simulink model "joystick_ctrl"  (Simulink 6.4)
settings: Solver=FixedStepDiscrete  SolverMode=SingleTasking  StartTime=0  StopTime=inf  FixedStep=0.001  RelTol=1e-3
PreLoadFcn:
  | load_logdata;
  | SoundList;
libraries: ecrobot_nxt_lib x10, simulink x4
CloseFcn:
  | rtwprivate ssgencode ModelCloseRequest TestBluetooth
settings Model: Creator=banno  LastModifiedBy=tchikama  CovPath=/Joystick_app  CovMetricSettings=dcmtrw  ProdHWDeviceType=ARM7
settings DataIOCC: SaveOutput=off  SignalLogging=off  SaveTime=off
settings OptimizationCC: InlineParams=on  InlineInvariantSignals=on  RollThreshold=2  StateBitsets=on  DataBitsets=on  UseTempVars=on  InitFltsAndDblsToZero=off  NoFixptDivByZeroProtection=on  EfficientFloat2IntCast=on  OptimizeModelRefInitCode=on  LifeSpan=1
settings DebuggingCC: ConsistencyChecking=warning  SignalInfNanChecking=warning  ReadBeforeWriteMsg=DisableAll  WriteAfterWriteMsg=DisableAll  WriteAfterReadMsg=DisableAll  AlgebraicLoopMsg=error  CheckExecutionContextPreStartOutputMsg=on  CheckExecutionContextRuntimeOutputMsg=on  SolverPrmCheckMsg=none  SingleTaskRateTransMsg=warning  TasksWithSamePriorityMsg=none  IntegerOverflowMsg=error  ParameterPrecisionLossMsg=none  UnconnectedInputMsg=error  UnconnectedOutputMsg=error  UnconnectedLineMsg=error  UniqueDataStoreMsg=error  BusObjectLabelMismatch=error  RootOutportRequireBusObject=error  ModelReferenceIOMsg=warning  ModelReferenceVersionMismatchMessage=warning  ModelReferenceIOMismatchMessage=warning
settings HardwareCC: ProdIntDivRoundTo=Zero  ProdEndianess=LittleEndian  ProdHWDeviceType=ARM7  TargetHWDeviceType=32-bit Generic
settings ModelReferenceCC: ModelReferenceNumInstancesAllowed=Single
settings RTWCC: SystemTargetFile=ert.tlc  GenCodeOnly=on  GenerateMakefile=off  TemplateMakefile=ert_default_tmf  Description=Real-Time Workshop Embedded Coder (no auto configuration)  GenerateReport=on  RTWVerbose=off  ProcessScript=ert_make_rtw_hook  IncludeHyperlinkInReport=on  LaunchReport=on
settings CodeAppCC: ForceParamTrailComments=on  IgnoreCustomStorageClasses=off  SFDataObjDesc=on  PrefixModelToSubsysFcnNames=off  CustomSymbolStrGlobalVar=rt$N$M  CustomSymbolStrType=$N$M  CustomSymbolStrFcn=$N$M$F  CustomSymbolStrMacro=$N$M  InsertBlockDesc=on
settings ERTTargetCC: TargetFcnLib=ansi_tfl_tmw.mat  GenFloatMathFcnCalls=GNU  IncludeMdlTerminateFcn=off  SuppressErrorStatus=on  IncludeERTFirstTime=on  SupportAbsoluteTime=off  SupportNonFinite=off  SupportComplex=off  InlinedParameterPlacement=NonHierarchical  RootIOFormat=Structure reference  ERTCustomFileTemplate=example_file_process.tlc  InitialValueSource=Model

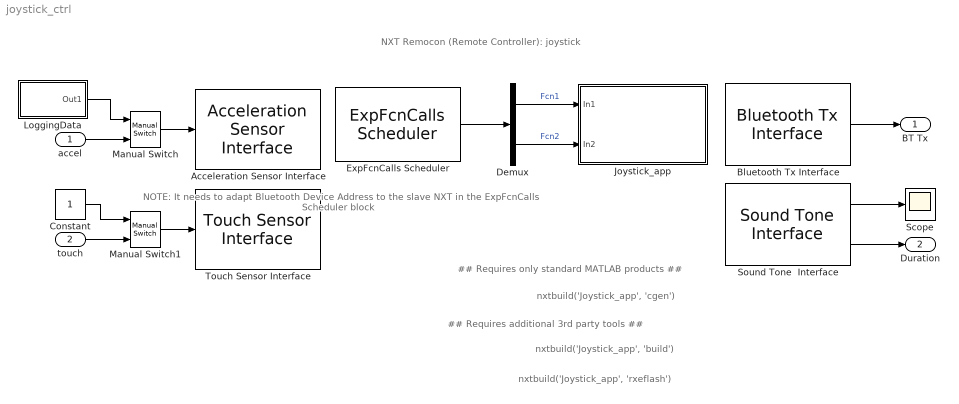
== system joystick_ctrl ==
  note: nxtbuild('Joystick_app', 'build')
  note: nxtbuild('Joystick_app', 'rxeflash')
  note: nxtbuild('Joystick_app', 'cgen')
  note: ## Requires only standard MATLAB products ##
  note: ## Requires additional 3rd party tools ##
  note: NXT Remocon (Remote Controller): joystick
  note: NOTE: It needs to adapt Bluetooth Device Address to the slave NXT
      | in the ExpFcnCalls Scheduler block
  accel : Inport  DataType=int16
  touch : Inport  Port=2  OutDataType=fixdt(1,16,0)  OutScaling=[]
  Acceleration Sensor Interface : ecrobot_nxt_lib/Acceleration Sensor Interface  SystemSampleTime=-1  ip=S1
  Bluetooth Tx Interface : ecrobot_nxt_lib/Bluetooth Tx Interface  SystemSampleTime=-1
  Constant : Constant  Value=1  OutDataTypeMode=uint8  OutDataType=sfix(16)  ConRadixGroup=Use specified scaling  OutScaling=2^0  SampleTime=inf  FramePeriod=inf
  Demux : Demux  Outputs=2
  ExpFcnCalls Scheduler : ecrobot_nxt_lib/ExpFcnCalls Scheduler  Priority=1  fcname='Fcn1','Fcn2'  fctrigger=[10 50]  ts=0.001  platform=OSEK  stacksize=[512 512]  bd_mode=Master  bd_addr='00', '16', '53', '04', '7E', '2D', '00'
  Joystick_app : Subsystem
      mask Display: image(imread('joystick_ctrl.JPG'))
  LoggingData : Subsystem
  Manual Switch : simulink/Signal Routing/Manual Switch  SystemSampleTime=-1  sw=1  action=0
  Manual Switch1 : simulink/Signal Routing/Manual Switch  SystemSampleTime=-1  sw=1  action=0
  Scope : Scope
      settings: TimeRange=20  YMin=0  YMax=1600
  Sound Tone  Interface : ecrobot_nxt_lib/Sound Tone  Interface  Priority=2  SystemSampleTime=-1
  Touch Sensor Interface : ecrobot_nxt_lib/Touch Sensor Interface  SystemSampleTime=-1  ip=S2
  BT Tx : Outport
  Duration : Outport  Port=2
  wires:
  ExpFcnCalls Scheduler/1 -> Demux/1
  Demux/1 -> Joystick_app/1(In1)  "Fcn1"
  Bluetooth Tx Interface/1 -> BT Tx/1
  Manual Switch/1 -> Acceleration Sensor Interface/1
  accel/1 -> Manual Switch/2
  LoggingData/1(Out1) -> Manual Switch/1
  Manual Switch1/1 -> Touch Sensor Interface/1
  touch/1 -> Manual Switch1/2
  Constant/1 -> Manual Switch1/1
  Sound Tone  Interface/1 -> Scope/1
  Sound Tone  Interface/2 -> Duration/1
  Demux/2 -> Joystick_app/2(In2)  "Fcn2"

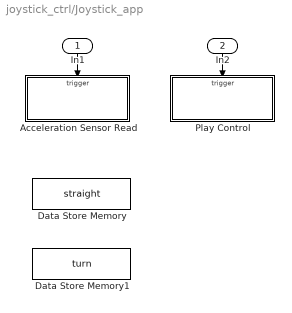
== system joystick_ctrl/Joystick_app ==
  In1 : Inport  Orientation=down
  In2 : Inport  Orientation=down  Port=2
  Acceleration Sensor Read : Subsystem  TreatAsAtomicUnit=on
  Data Store Memory : DataStoreMemory  DataStoreName=straight  ReadBeforeWriteMsg=warning  WriteAfterWriteMsg=warning  WriteAfterReadMsg=warning  InitialValue=0  DataType=int8
      settings: AttributesFormatString=DataType=%<DataType>
  Data Store Memory1 : DataStoreMemory  DataStoreName=turn  ReadBeforeWriteMsg=warning  WriteAfterWriteMsg=warning  WriteAfterReadMsg=warning  InitialValue=0  DataType=int8
      settings: AttributesFormatString=DataType=%<DataType>
  Play Control : Subsystem  TreatAsAtomicUnit=on
  wires:
  In1/1 -> Acceleration Sensor Read/Trigger
  In2/1 -> Play Control/Trigger

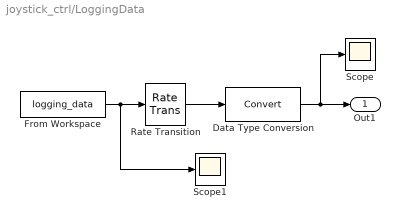
== system joystick_ctrl/LoggingData ==
  Data Type Conversion : DataTypeConversion  OutDataTypeMode=int16
  From Workspace : FromWorkspace  VariableName=logging_data  SampleTime=0.01  Interpolate=off  OutputAfterFinalValue=Holding final value
  Rate Transition : RateTransition  Integrity=off  OutPortSampleTime=0.001
  Scope : Scope
      settings: TimeRange=20  YMin=-300  YMax=300
  Scope1 : Scope
      settings: TimeRange=20  YMin=-300  YMax=300  SaveName=ScopeData4
  Out1 : Outport
  wires:
  From Workspace/1 -> Rate Transition/1, Scope1/1
  Data Type Conversion/1 -> Out1/1, Scope/1
  Rate Transition/1 -> Data Type Conversion/1

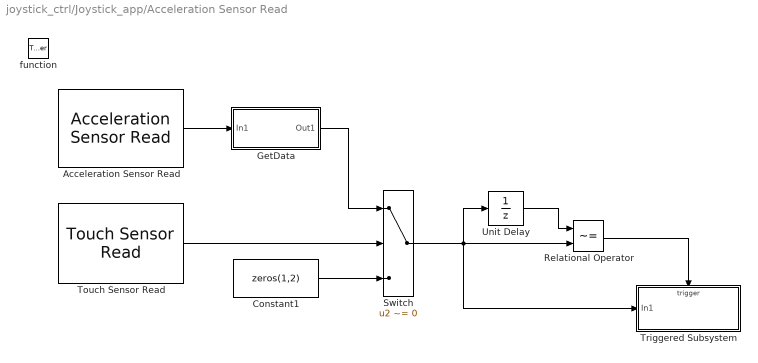
== system joystick_ctrl/Joystick_app/Acceleration Sensor Read ==
  function : TriggerPort  TriggerType=function-call
  Acceleration Sensor Read : ecrobot_nxt_lib/Acceleration Sensor Read  ip=S1
  Constant1 : Constant  Value=zeros(1,2)  OutDataTypeMode=uint8  OutDataType=sfix(16)  ConRadixGroup=Use specified scaling  OutScaling=2^0  SampleTime=-1  FramePeriod=inf
  GetData : Subsystem
  Relational Operator : RelationalOperator  Operator=~=  LogicOutDataTypeMode=Boolean
  Switch : Switch  Criteria=u2 ~= 0
  Touch Sensor Read : ecrobot_nxt_lib/Touch Sensor Read  SystemSampleTime=-1  ip=S2
  Triggered Subsystem : Subsystem  TreatAsAtomicUnit=on
  Unit Delay : UnitDelay  SampleTime=-1
  wires:
  Touch Sensor Read/1 -> Switch/2
  Constant1/1 -> Switch/3
  Acceleration Sensor Read/1 -> GetData/1(In1)
  GetData/1(Out1) -> Switch/1
  Relational Operator/1 -> Triggered Subsystem/Trigger
  Unit Delay/1 -> Relational Operator/1
  Switch/1 -> Relational Operator/2, Unit Delay/1, Triggered Subsystem/1(In1)

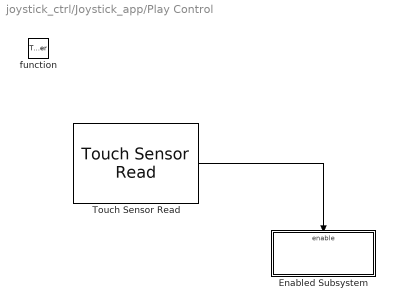
== system joystick_ctrl/Joystick_app/Play Control ==
  function : TriggerPort  TriggerType=function-call
  Enabled Subsystem : Subsystem  TreatAsAtomicUnit=on
  Touch Sensor Read : ecrobot_nxt_lib/Touch Sensor Read  SystemSampleTime=-1  ip=S2
  wires:
  Touch Sensor Read/1 -> Enabled Subsystem/Enable

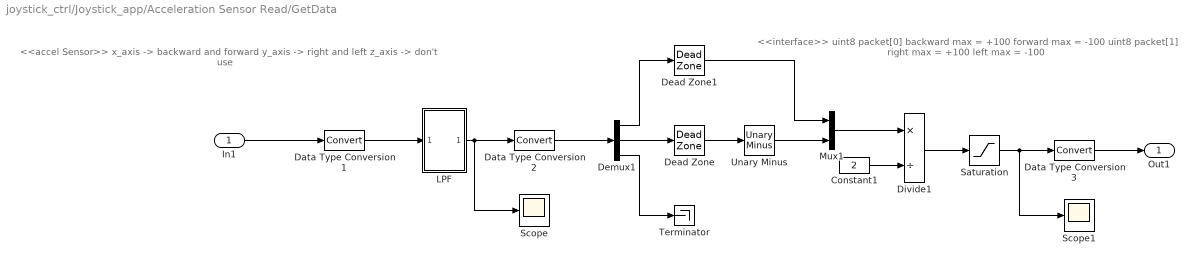
== system joystick_ctrl/Joystick_app/Acceleration Sensor Read/GetData ==
  note: <<interface>>
      | uint8 packet[0]
      |   backward max = +100
      |   forward max = -100
      | uint8 packet[1]
      |   right max = +100
      |   left max = -100
  note: <<accel Sensor>>
      | x_axis -> backward and forward
      | y_axis -> right and left
      | z_axis -> don't use
  In1 : Inport  OutDataType=fixdt(1,16,0)  OutScaling=[]
  Constant1 : Constant  Value=2  OutDataTypeMode=int16  OutDataType=sfix(16)  ConRadixGroup=Use specified scaling  OutScaling=2^0  SampleTime=inf  FramePeriod=inf
  Data Type Conversion1 : DataTypeConversion  OutDataTypeMode=single
      settings: AttributesFormatString=Round = %<RndMeth>
  Data Type Conversion2 : DataTypeConversion  OutDataTypeMode=int16  RndMeth=Simplest
      settings: AttributesFormatString=Round = %<RndMeth>
  Data Type Conversion3 : DataTypeConversion  OutDataTypeMode=uint8  RndMeth=Simplest
      settings: AttributesFormatString=Round = %<RndMeth>
  Dead Zone : DeadZone  LowerValue=-10  UpperValue=10  SaturateOnIntegerOverflow=on
  Dead Zone1 : DeadZone  LowerValue=-20  UpperValue=20  SaturateOnIntegerOverflow=on
  Demux1 : Demux  Outputs=3
  Divide1 : Product  Inputs=*/  OutScaling=2^-10  RndMeth=Simplest
  LPF : Subsystem
  Mux1 : Mux  Inputs=2
  Saturation : Saturate  UpperLimit=100  LowerLimit=-100  LinearizeAsGain=off
  Scope : Scope
      settings: TimeRange=20  YMin=-300  YMax=300  SaveName=ScopeData2
  Scope1 : Scope
      settings: TimeRange=20  YMin=-100  YMax=100  SaveName=ScopeData3
  Terminator : Terminator
  Unary Minus : simulink/Math Operations/Unary Minus  DoSatur=off
  Out1 : Outport  OutDataType=fixdt(1,16,0)  OutScaling=[]
  wires:
  Data Type Conversion3/1 -> Out1/1
  Saturation/1 -> Data Type Conversion3/1, Scope1/1
  Data Type Conversion2/1 -> Demux1/1
  Demux1/3 -> Terminator/1
  Demux1/2 -> Dead Zone/1
  Demux1/1 -> Dead Zone1/1
  Dead Zone/1 -> Unary Minus/1
  Dead Zone1/1 -> Mux1/1
  In1/1 -> Data Type Conversion1/1
  LPF/1(Out1) -> Data Type Conversion2/1, Scope/1
  Data Type Conversion1/1 -> LPF/1(In1)
  Unary Minus/1 -> Mux1/2
  Mux1/1 -> Divide1/1
  Divide1/1 -> Saturation/1
  Constant1/1 -> Divide1/2

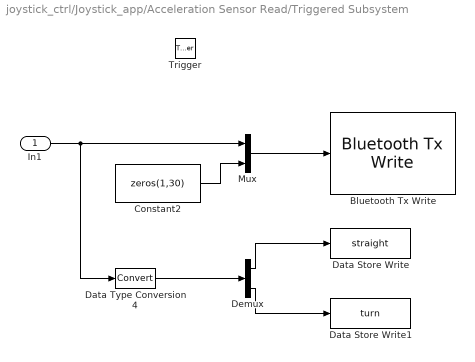
== system joystick_ctrl/Joystick_app/Acceleration Sensor Read/Triggered Subsystem ==
  In1 : Inport
  Trigger : TriggerPort  TriggerType=either
  Bluetooth Tx Write : ecrobot_nxt_lib/Bluetooth Tx Write
  Constant2 : Constant  Value=zeros(1,30)  OutDataTypeMode=uint8  OutDataType=sfix(16)  ConRadixGroup=Use specified scaling  OutScaling=2^0  SampleTime=-1  FramePeriod=inf
  Data Store Write : DataStoreWrite  DataStoreName=straight  SampleTime=-1
  Data Store Write1 : DataStoreWrite  DataStoreName=turn  SampleTime=-1
  Data Type Conversion4 : DataTypeConversion  OutDataTypeMode=int8  RndMeth=Simplest
      settings: AttributesFormatString=Round = %<RndMeth>
  Demux : Demux  Outputs=2
  Mux : Mux  Inputs=2
  wires:
  In1/1 -> Data Type Conversion4/1, Mux/1
  Data Type Conversion4/1 -> Demux/1
  Demux/1 -> Data Store Write/1
  Demux/2 -> Data Store Write1/1
  Constant2/1 -> Mux/2
  Mux/1 -> Bluetooth Tx Write/1

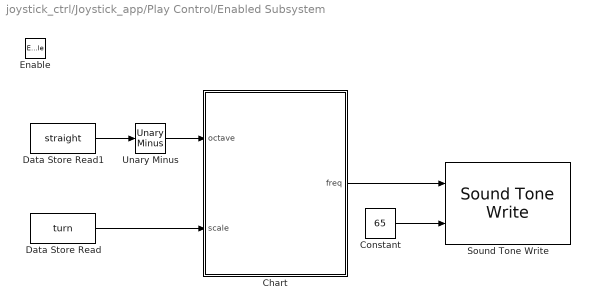
== system joystick_ctrl/Joystick_app/Play Control/Enabled Subsystem ==
  Enable : EnablePort
  Chart : Stateflow chart
  Constant : Constant  Value=65  OutDataType=sfix(16)  ConRadixGroup=Use specified scaling  OutScaling=2^0  SampleTime=-1  FramePeriod=inf
  Data Store Read : DataStoreRead  DataStoreName=turn  SampleTime=-1
  Data Store Read1 : DataStoreRead  DataStoreName=straight  SampleTime=-1
  Sound Tone Write : ecrobot_nxt_lib/Sound Tone Write
  Unary Minus : simulink/Math Operations/Unary Minus  DoSatur=off
  wires:
  Data Store Read/1 -> Chart/2(scale)
  Data Store Read1/1 -> Unary Minus/1
  Chart/1(freq) -> Sound Tone Write/1
  Constant/1 -> Sound Tone Write/2
  Unary Minus/1 -> Chart/1(octave)

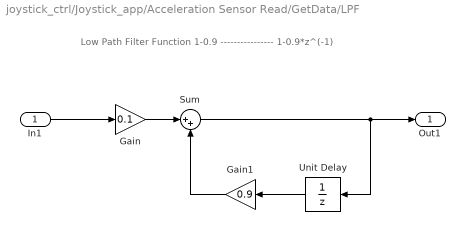
== system joystick_ctrl/Joystick_app/Acceleration Sensor Read/GetData/LPF ==
  note: Low Path Filter Function
      |       1-0.9
      |          ----------------
      |          1-0.9*z^(-1)
  In1 : Inport
  Gain : Gain  Gain=0.1
  Gain1 : Gain  Orientation=left  Gain=0.9
  Sum : Sum  Inputs=|++
  Unit Delay : UnitDelay  Orientation=left  SampleTime=-1
  Out1 : Outport
  wires:
  In1/1 -> Gain/1
  Unit Delay/1 -> Gain1/1
  Gain/1 -> Sum/1
  Sum/1 -> Out1/1, Unit Delay/1
  Gain1/1 -> Sum/2

== stateflow chart Joystick_app/Play Control/Enabled Subsystem/Chart ==
  state zone4(data) [function]
    (default) -> (junction 16)
    (junction 16) -> (junction 17) [order 1] : [data > 80]
    (junction 16) -> (junction 18) [order 2]
    (junction 18) -> (junction 19) [order 1] : [data >= -20]
    (junction 18) -> (junction 20) [order 2]
    (junction 20) -> (junction 21) [order 1] : [data > -80]
    (junction 20) -> (junction 22) [order 2] : {
        | zone=0;
        | }
    (junction 21) -> (junction 23) : {
        | zone=1;
        | }
    (junction 19) -> (junction 24) : {
        | zone=2;
        | }
    (junction 17) -> (junction 25) : {
        | zone=3;
        | }
    (junction 25) -> (junction 24)
    (junction 24) -> (junction 23)
    (junction 23) -> (junction 22)
    (junction 22) -> (junction 26)
  state zone8(data) [function]
    (junction 36) -> (junction 35) [order 1] : [data > -30]
    (junction 38) -> (junction 37) [order 1] : [data >= -10]
    (junction 38) -> (junction 36) [order 2]
    (junction 9) -> (junction 5)
    (junction 6) -> (junction 7)
    (junction 7) -> (junction 8)
    (default) -> (junction 15)
    (junction 10) -> (junction 8) : {
        | zone=5;
        | }
    (junction 15) -> (junction 14) [order 1] : [data > 80]
    (junction 11) -> (junction 10) [order 1] : [data > 30]
    (junction 12) -> (junction 7) : {
        | zone=6;
        | }
    (junction 13) -> (junction 11) [order 2]
    (junction 13) -> (junction 12) [order 1] : [data > 60]
    (junction 14) -> (junction 6) : {
        | zone=7;
        | }
    (junction 27) -> (junction 9)
    (junction 28) -> (junction 27)
    (junction 29) -> (junction 28)
    (junction 30) -> (junction 29)
    (junction 8) -> (junction 30)
    (junction 32) -> (junction 9) [order 2] : {
        | zone=0;
        | }
    (junction 31) -> (junction 27) : {
        | zone=1;
        | }
    (junction 33) -> (junction 28) : {
        | zone=2;
        | }
    (junction 35) -> (junction 29) : {
        | zone=3;
        | }
    (junction 37) -> (junction 30) : {
        | zone=4;
        | }
    (junction 32) -> (junction 31) [order 1] : [data > -80]
    (junction 34) -> (junction 32) [order 2]
    (junction 34) -> (junction 33) [order 1] : [data > -60]
    (junction 36) -> (junction 34) [order 2]
    (junction 15) -> (junction 13) [order 2]
    (junction 11) -> (junction 38) [order 2]
  (default) -> (junction 39) : {
      | zone8(scale);
      | scale_index=zone;
      | zone4(octave);
      | octave_index=zone;
      | freq=frequency[octave_index][scale_index];
      | }
  data: data function_input double; data function_input double; octave input int16; scale input int16; octave_index local uint8; scale_index local uint8; freq output uint32; zone local uint8; frequency parameter double
